simulink library "vhit_control_library"  (R2023a)
settings: Solver=VariableStepAuto  StartTime=0.0  StopTime=10.0  RelTol=1e-3
undefined symbols (not defined in the file): bit, cstElctSpdMaxVal, cstSlowTaskSampTime, parDirCurrMaxVal, parElctSpdMaxVal, parFluxObsFiltCoef, parQdrtCurrMaxVal, parRefSpdFallSlewRate, parRefSpdRisSlewRate, PolePairNum
libraries: lib_conversion x90, lib_square_root x11, lib_dynamic_saturator x9, lib_resettable_unit_delay x2, lib_fault_definiteness x1, lib_angle_mapper x1, lib_cart_to_polar_coor_transformer x1, lib_clarke_transform x1, lib_configurable_parameter x1, lib_current_control_decoupling x1, lib_derating_reference_speed_limiter x1, lib_discrete_time_integrator x1
(part 2 of 3)

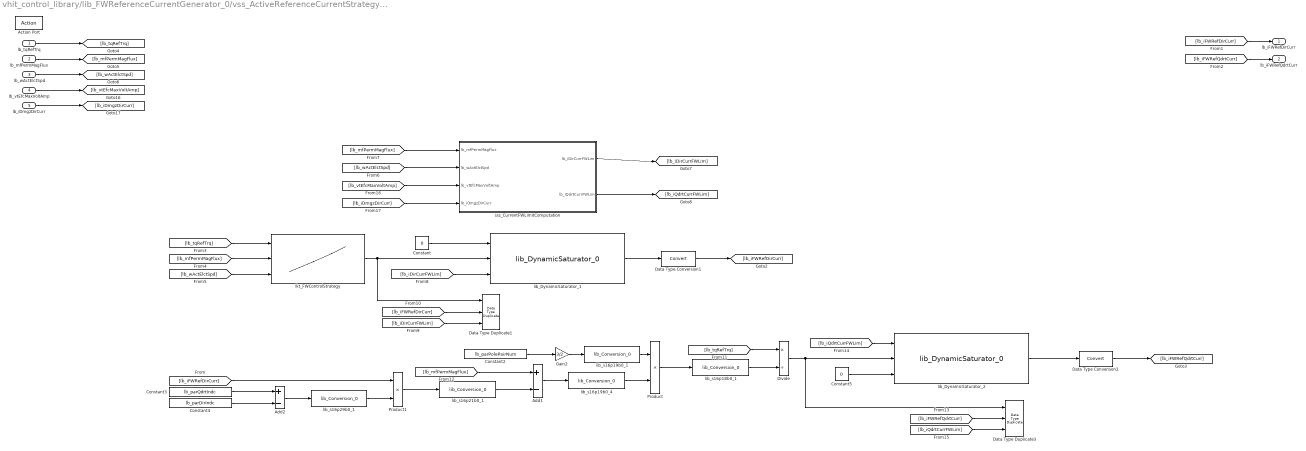
== system vhit_control_library/lib_FWReferenceCurrentGenerator_0/vss_ActiveReferenceCurrentStrategy/vss_FieldWeakeningStrategy/ias_FWControlStrategy ==
  lb_tqRefTrq : Inport
  lb_mfPermMagFlux : Inport  Port=2
  lb_wActElctSpd : Inport  Port=3
  lb_vtEfcMaxVoltAmp : Inport  Port=4
  lb_iDmgzDirCurr : Inport  Port=5
  Action Port : ActionPort
  Add1 : Sum  Inputs=+-  OutDataTypeStr=Inherit: Inherit via back propagation
  Add2 : Sum  Inputs=+-  OutDataTypeStr=Inherit: Inherit via back propagation
  Constant : Constant  Value=0  OutDataTypeStr=Inherit: Inherit via back propagation
  Constant2 : Constant  Value=lb_parPolePairNum
  Constant3 : Constant  Value=lb_parQdrtIndc
  Constant4 : Constant  Value=lb_parDirIndc
  Constant5 : Constant  Value=0  OutDataTypeStr=Inherit: Inherit via back propagation
  Data Type Duplicate1 : DataTypeDuplicate  NumInputPorts=3
  Data Type Duplicate3 : DataTypeDuplicate  NumInputPorts=3
  Data Type Conversion1 : DataTypeConversion  SaturateOnIntegerOverflow=off  RndMeth=Floor
  Data Type Conversion2 : DataTypeConversion  SaturateOnIntegerOverflow=off  RndMeth=Floor
  Divide : Product  Inputs=*/  OutDataTypeStr=Inherit: Inherit via back propagation
  Gain2 : Gain  Gain=3/2  OutDataTypeStr=Inherit: Inherit via back propagation
  Product : Product  OutDataTypeStr=Inherit: Inherit via back propagation
  Product1 : Product  OutDataTypeStr=Inherit: Inherit via back propagation
  lib_DynamicSaturator_1 : lib_dynamic_saturator/lib_DynamicSaturator_0
  lib_DynamicSaturator_2 : lib_dynamic_saturator/lib_DynamicSaturator_0
  lib_s16p18b0_1 : lib_conversion/lib_Conversion_0  lb_parDataType=fixdt(1,16,2^-18,0)  lb_parOutpMaxVal=[]  lb_parOutpMinVal=[]  lb_parSatFlag=off
  lib_s16p19b0_1 : lib_conversion/lib_Conversion_0  lb_parDataType=fixdt(0,16,10^-3,0)  lb_parOutpMaxVal=[]  lb_parOutpMinVal=[]  lb_parSatFlag=off
  lib_s16p19b0_4 : lib_conversion/lib_Conversion_0  lb_parDataType=fixdt(1,16,2^-19,0)  lb_parOutpMaxVal=[]  lb_parOutpMinVal=[]  lb_parSatFlag=off
  lib_s16p21b0_1 : lib_conversion/lib_Conversion_0  lb_parDataType=fixdt(1,16,2^-21,0)  lb_parOutpMaxVal=[]  lb_parOutpMinVal=[]  lb_parSatFlag=off
  lib_s16p29b0_1 : lib_conversion/lib_Conversion_0  lb_parDataType=fixdt(1,16,2^-29,0)  lb_parOutpMaxVal=[]  lb_parOutpMinVal=[]  lb_parSatFlag=off
  lkt_FWControlStrategy : Lookup_n-D  NumberOfTableDimensions=3  BreakpointsForDimension1=lb_parFWTrqData  BreakpointsForDimension2=lb_parFWPermMagFluxData  BreakpointsForDimension3=lb_parFWElctSpdData  BeginIndexSearchUsingPreviousIndexResult=on  Table=lb_parFW3DLktMtrx  ExtrapMethod=Clip  InternalRulePriority=Speed  OutDataTypeStr=Inherit: Inherit via back propagation  RndMeth=Simplest  InputSameDT=off
      settings: InputPortMap=u0,u1,u2
  sss_CurrentFWLimitComputation : Subsystem
  lb_iFWRefDirCurr : Outport
  lb_iFWRefQdrtCurr : Outport  Port=2
  wires:
  Constant2/1 -> Gain2/1
  Gain2/1 -> lib_s16p19b0_1/1
  lib_s16p19b0_1/1 -> Product/1
  [lb_wActElctSpd] -> sss_CurrentFWLimitComputation/2(lb_wActElctSpd)
  sss_CurrentFWLimitComputation/2(lb_iQdrtCurrFWLim) -> [lb_iQdrtCurrFWLim]
  [lb_mfPermMagFlux] -> sss_CurrentFWLimitComputation/1(lb_mfPermMagFlux)
  sss_CurrentFWLimitComputation/1(lb_iDirCurrFWLim) -> [lb_iDirCurrFWLim]
  Constant/1 -> lib_DynamicSaturator_1/1
  [lb_iDirCurrFWLim] -> lib_DynamicSaturator_1/3
  [lb_iFWRefDirCurr] -> lb_iFWRefDirCurr/1
  [lb_iFWRefQdrtCurr] -> lb_iFWRefQdrtCurr/1
  lb_mfPermMagFlux/1 -> [lb_mfPermMagFlux]
  lb_tqRefTrq/1 -> [lb_tqRefTrq]
  lb_wActElctSpd/1 -> [lb_wActElctSpd]
  [lb_tqRefTrq] -> lkt_FWControlStrategy/1
  [lb_mfPermMagFlux] -> lkt_FWControlStrategy/2
  [lb_wActElctSpd] -> lkt_FWControlStrategy/3
  lkt_FWControlStrategy/1 -> Data Type Duplicate1/1, lib_DynamicSaturator_1/2
  [lb_iFWRefDirCurr] -> Data Type Duplicate1/2
  [lb_iQdrtCurrFWLim] -> Data Type Duplicate3/3
  Constant5/1 -> lib_DynamicSaturator_2/3
  [lb_iQdrtCurrFWLim] -> lib_DynamicSaturator_2/1
  Data Type Conversion2/1 -> [lb_iFWRefQdrtCurr]
  lib_DynamicSaturator_2/1 -> Data Type Conversion2/1
  [lb_iFWRefQdrtCurr] -> Data Type Duplicate3/2
  Divide/1 -> Data Type Duplicate3/1, lib_DynamicSaturator_2/2
  [lb_iFWRefDirCurr] -> Product1/1
  lib_s16p19b0_4/1 -> Product/2
  Add1/1 -> lib_s16p19b0_4/1
  Add2/1 -> lib_s16p29b0_1/1
  Constant4/1 -> Add2/2
  Constant3/1 -> Add2/1
  Product1/1 -> lib_s16p21b0_1/1
  lib_s16p18b0_1/1 -> Divide/2
  [lb_mfPermMagFlux] -> Add1/1
  lib_s16p29b0_1/1 -> Product1/2
  Product/1 -> lib_s16p18b0_1/1
  lib_s16p21b0_1/1 -> Add1/2
  [lb_tqRefTrq] -> Divide/1
  lib_DynamicSaturator_1/1 -> Data Type Conversion1/1
  Data Type Conversion1/1 -> [lb_iFWRefDirCurr]
  [lb_iDirCurrFWLim] -> Data Type Duplicate1/3
  lb_vtEfcMaxVoltAmp/1 -> [lb_vtEfcMaxVoltAmp]
  lb_iDmgzDirCurr/1 -> [lb_iDmgzDirCurr]
  [lb_vtEfcMaxVoltAmp] -> sss_CurrentFWLimitComputation/3(lb_vtEfcMaxVoltAmp)
  [lb_iDmgzDirCurr] -> sss_CurrentFWLimitComputation/4(lb_iDmgzDirCurr)

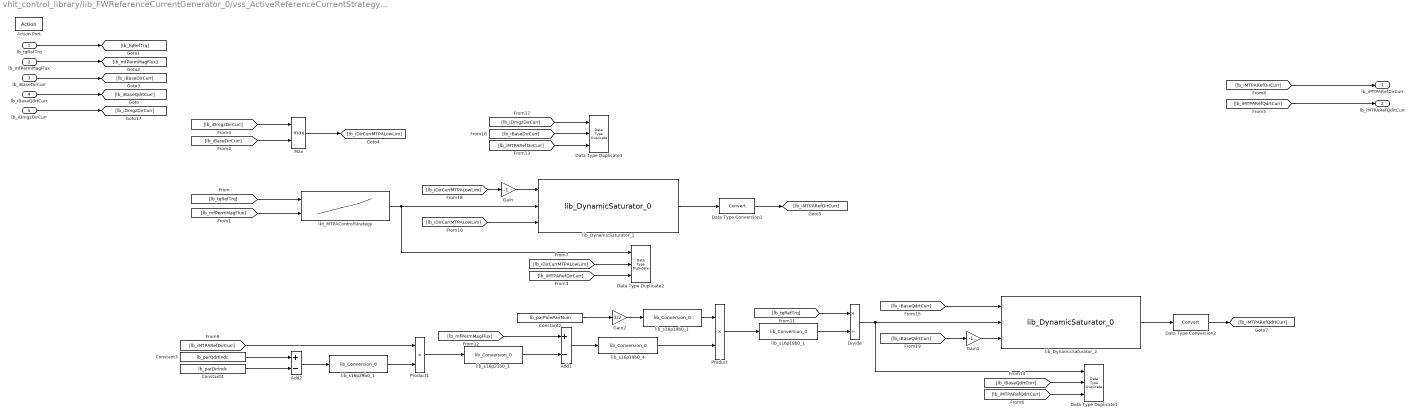
== system vhit_control_library/lib_FWReferenceCurrentGenerator_0/vss_ActiveReferenceCurrentStrategy/vss_FieldWeakeningStrategy/ias_MTPAControlStrategy ==
  lb_tqRefTrq : Inport
  lb_mfPermMagFlux : Inport  Port=2
  lb_iBaseDirCurr : Inport  Port=3
  lb_iBaseQdrtCurr : Inport  Port=4
  lb_iDmgzDirCurr : Inport  Port=5
  Action Port : ActionPort
  Add1 : Sum  Inputs=+-  OutDataTypeStr=Inherit: Inherit via back propagation
  Add2 : Sum  Inputs=+-  OutDataTypeStr=Inherit: Inherit via back propagation
  Constant2 : Constant  Value=lb_parPolePairNum
  Constant3 : Constant  Value=lb_parQdrtIndc
  Constant4 : Constant  Value=lb_parDirIndc
  Data Type Duplicate1 : DataTypeDuplicate  NumInputPorts=3
  Data Type Duplicate2 : DataTypeDuplicate  NumInputPorts=3
  Data Type Duplicate3 : DataTypeDuplicate  NumInputPorts=3
  Data Type Conversion1 : DataTypeConversion  SaturateOnIntegerOverflow=off  RndMeth=Floor
  Data Type Conversion2 : DataTypeConversion  SaturateOnIntegerOverflow=off  RndMeth=Floor
  Divide : Product  Inputs=*/  OutDataTypeStr=Inherit: Inherit via back propagation
  Gain : Gain  Gain=-1  OutDataTypeStr=Inherit: Inherit via back propagation
  Gain1 : Gain  Gain=-1  OutDataTypeStr=Inherit: Inherit via back propagation
  Gain2 : Gain  Gain=3/2  OutDataTypeStr=Inherit: Inherit via back propagation
  Max : MinMax  Function=max  Inputs=2  OutDataTypeStr=Inherit: Inherit via back propagation
  Product : Product  OutDataTypeStr=Inherit: Inherit via back propagation
  Product1 : Product  OutDataTypeStr=Inherit: Inherit via back propagation
  lib_DynamicSaturator_1 : lib_dynamic_saturator/lib_DynamicSaturator_0
  lib_DynamicSaturator_2 : lib_dynamic_saturator/lib_DynamicSaturator_0
  lib_s16p18b0_1 : lib_conversion/lib_Conversion_0  lb_parDataType=fixdt(1,16,2^-18,0)  lb_parOutpMaxVal=[]  lb_parOutpMinVal=[]  lb_parSatFlag=off
  lib_s16p19b0_1 : lib_conversion/lib_Conversion_0  lb_parDataType=fixdt(0,16,10^-3,0)  lb_parOutpMaxVal=[]  lb_parOutpMinVal=[]  lb_parSatFlag=off
  lib_s16p19b0_4 : lib_conversion/lib_Conversion_0  lb_parDataType=fixdt(1,16,2^-19,0)  lb_parOutpMaxVal=[]  lb_parOutpMinVal=[]  lb_parSatFlag=off
  lib_s16p21b0_1 : lib_conversion/lib_Conversion_0  lb_parDataType=fixdt(1,16,2^-21,0)  lb_parOutpMaxVal=[]  lb_parOutpMinVal=[]  lb_parSatFlag=off
  lib_s16p29b0_1 : lib_conversion/lib_Conversion_0  lb_parDataType=fixdt(1,16,2^-29,0)  lb_parOutpMaxVal=[]  lb_parOutpMinVal=[]  lb_parSatFlag=off
  lkt_MTPAControlStrategy : Lookup_n-D  BreakpointsForDimension1=lb_parMTPATrqData  BreakpointsForDimension2=lb_parMTPAPermMagFluxData  BeginIndexSearchUsingPreviousIndexResult=on  Table=lb_parMTPA2DLktMtrx  ExtrapMethod=Clip  InternalRulePriority=Speed  OutDataTypeStr=Inherit: Inherit via back propagation  RndMeth=Simplest  SaturateOnIntegerOverflow=on  InputSameDT=off
      settings: InputPortMap=u0,u1
  lb_iMTPARefDirCurr : Outport
  lb_iMTPARefQdrtCurr : Outport  Port=2
  wires:
  lib_s16p19b0_1/1 -> Product/1
  Gain2/1 -> lib_s16p19b0_1/1
  lb_tqRefTrq/1 -> [lb_tqRefTrq]
  lb_mfPermMagFlux/1 -> [lb_mfPermMagFlux]
  [lb_tqRefTrq] -> lkt_MTPAControlStrategy/1
  [lb_mfPermMagFlux] -> lkt_MTPAControlStrategy/2
  lkt_MTPAControlStrategy/1 -> lib_DynamicSaturator_1/2, Data Type Duplicate2/1
  [lb_iDirCurrMTPALowLim] -> Gain/1
  lib_DynamicSaturator_1/1 -> Data Type Conversion1/1
  [lb_iMTPARefDirCurr] -> lb_iMTPARefDirCurr/1
  [lb_iMTPARefQdrtCurr] -> lb_iMTPARefQdrtCurr/1
  Data Type Conversion1/1 -> [lb_iMTPARefDirCurr]
  [lb_iMTPARefDirCurr] -> Data Type Duplicate2/3
  [lb_iDirCurrMTPALowLim] -> Data Type Duplicate2/2
  Product/1 -> lib_s16p18b0_1/1
  lib_s16p19b0_4/1 -> Product/2
  Add1/1 -> lib_s16p19b0_4/1
  lib_s16p21b0_1/1 -> Add1/2
  lib_s16p18b0_1/1 -> Divide/2
  lib_s16p29b0_1/1 -> Product1/2
  Product1/1 -> lib_s16p21b0_1/1
  [lb_tqRefTrq] -> Divide/1
  [lb_mfPermMagFlux] -> Add1/1
  [lb_iMTPARefDirCurr] -> Product1/1
  Constant3/1 -> Add2/1
  Constant2/1 -> Gain2/1
  Constant4/1 -> Add2/2
  Add2/1 -> lib_s16p29b0_1/1
  [lb_iBaseQdrtCurr] -> Gain1/1
  Data Type Conversion2/1 -> [lb_iMTPARefQdrtCurr]
  lib_DynamicSaturator_2/1 -> Data Type Conversion2/1
  [lb_iBaseQdrtCurr] -> lib_DynamicSaturator_2/1
  Divide/1 -> lib_DynamicSaturator_2/2, Data Type Duplicate1/1
  lb_iBaseDirCurr/1 -> [lb_iBaseDirCurr]
  lb_iBaseQdrtCurr/1 -> [lb_iBaseQdrtCurr]
  [lb_iMTPARefQdrtCurr] -> Data Type Duplicate1/3
  [lb_iBaseQdrtCurr] -> Data Type Duplicate1/2
  lb_iDmgzDirCurr/1 -> [lb_iDmgzDirCurr]
  [lb_iBaseDirCurr] -> Max/2
  [lb_iDmgzDirCurr] -> Max/1
  Max/1 -> [lb_iDirCurrMTPALowLim]
  [lb_iDirCurrMTPALowLim] -> lib_DynamicSaturator_1/3
  [lb_iMTPARefDirCurr] -> Data Type Duplicate3/3
  [lb_iBaseDirCurr] -> Data Type Duplicate3/2
  [lb_iDmgzDirCurr] -> Data Type Duplicate3/1
  Gain/1 -> lib_DynamicSaturator_1/1
  Gain1/1 -> lib_DynamicSaturator_2/3

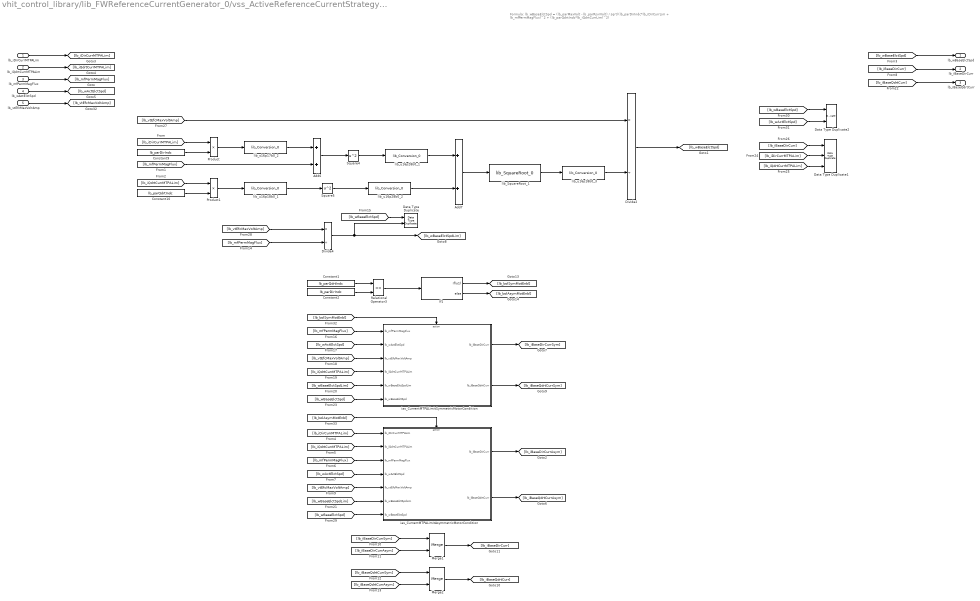
== system vhit_control_library/lib_FWReferenceCurrentGenerator_0/vss_ActiveReferenceCurrentStrategy/vss_FieldWeakeningStrategy/sss_BaseSpeedComputation ==
  note: Formula: lb_wBaseElctSpd = (lb_parMaxVolt - lb_parRsvrVolt) / sqrt((lb_parDirIndc*lb_iDirCurrLim + lb_mfPermMagFlux)^2 + (lb_parQdrtIndc*lb_iQdrtCurrLim)^2)
  lb_iDirCurrMTPALim : Inport
  lb_iQdrtCurrMTPALim : Inport  Port=2
  lb_mfPermMagFlux : Inport  Port=3
  lb_wActElctSpd : Inport  Port=4
  lb_vtEfcMaxVoltAmp : Inport  Port=5
  Add6 : Sum  OutDataTypeStr=Inherit: Same as first input
  Add7 : Sum  OutDataTypeStr=Inherit: Same as first input
  Constant1 : Constant  Value=lb_parQdrtIndc
  Constant10 : Constant  Value=lb_parQdrtIndc
  Constant2 : Constant  Value=lb_parDirIndc
  Constant9 : Constant  Value=lb_parDirIndc
  Data Type Duplicate : DataTypeDuplicate
  Data Type Duplicate1 : DataTypeDuplicate  NumInputPorts=3
  Data Type Duplicate2 : DataTypeDuplicate
  Divide2 : Product  Inputs=*/  OutDataTypeStr=Inherit: Inherit via back propagation
  Divide4 : Product  Inputs=*/  OutDataTypeStr=Inherit: Inherit via back propagation
  If1 : If  IfExpression=u1
  Merge1 : Merge
  Merge2 : Merge
  Product : Product  OutDataTypeStr=Inherit: Inherit via back propagation
  Product1 : Product  OutDataTypeStr=Inherit: Inherit via back propagation
  Relational Operator3 : RelationalOperator  Operator===  OutDataTypeStr=boolean  RndMeth=Simplest  InputSameDT=off
  Square4 : Math  Operator=square  SignedPower=on  OutDataTypeStr=Inherit: Inherit via back propagation
  Square5 : Math  Operator=square  SignedPower=on  OutDataTypeStr=Inherit: Inherit via back propagation
  ias_CurrentMTPALimitAsymmetricMotorCondition : Subsystem  TreatAsAtomicUnit=on
  ias_CurrentMTPALimitSymmetricMotorCondition : Subsystem  TreatAsAtomicUnit=on
  lib_SquareRoot_1 : lib_square_root/lib_SquareRoot_0  lb_parLktSize=128  lb_parInpDataType=uint16  lb_parOutpDataType=Inherit: Inherit via back propagation
  lib_s16p17b0_2 : lib_conversion/lib_Conversion_0  lb_parDataType=fixdt(1,16,2^-17,0)  lb_parOutpMaxVal=[]  lb_parOutpMinVal=[]  lb_parSatFlag=off
  lib_u16p18b0_1 : lib_conversion/lib_Conversion_0  lb_parDataType=fixdt(0,16,2^-18,0)  lb_parOutpMaxVal=[]  lb_parOutpMinVal=[]  lb_parSatFlag=off
  lib_u16p18b0_3 : lib_conversion/lib_Conversion_0  lb_parDataType=fixdt(0,16,2^-18,0)  lb_parOutpMaxVal=[]  lb_parOutpMinVal=[]  lb_parSatFlag=off
  lib_u16p28b0_1 : lib_conversion/lib_Conversion_0  lb_parDataType=fixdt(0,16,2^-28,0)  lb_parOutpMaxVal=[]  lb_parOutpMinVal=[]  lb_parSatFlag=off
  lib_u16p28b0_2 : lib_conversion/lib_Conversion_0  lb_parDataType=fixdt(0,16,2^-28,0)  lb_parOutpMaxVal=[]  lb_parOutpMinVal=[]  lb_parSatFlag=off
  lb_wBaseElctSpd : Outport
  lb_iBaseDirCurr : Outport  Port=2
  lb_iBaseQdrtCurr : Outport  Port=3
  wires:
  [lb_wBaseElctSpd] -> ias_CurrentMTPALimitAsymmetricMotorCondition/7(lb_wBaseElctSpd)
  [lb_wBaseElctSpd] -> ias_CurrentMTPALimitSymmetricMotorCondition/6(lb_wBaseElctSpd)
  [lb_wBaseElctSpdLim] -> ias_CurrentMTPALimitAsymmetricMotorCondition/6(lb_wBaseElctSpdLim)
  [lb_wBaseElctSpdLim] -> ias_CurrentMTPALimitSymmetricMotorCondition/5(lb_wBaseElctSpdLim)
  [lb_iQdrtCurrMTPALim] -> ias_CurrentMTPALimitSymmetricMotorCondition/4(lb_iQdrtCurrMTPALim)
  [lb_vtEfcMaxVoltAmp] -> ias_CurrentMTPALimitSymmetricMotorCondition/3(lb_vtEfcMaxVoltAmp)
  [lb_wActElctSpd] -> ias_CurrentMTPALimitSymmetricMotorCondition/2(lb_wActElctSpd)
  [lb_mfPermMagFlux] -> ias_CurrentMTPALimitSymmetricMotorCondition/1(lb_mfPermMagFlux)
  Merge2/1 -> [lb_iBaseQdrtCurr]
  [lb_iBaseQdrtCurrAsym] -> Merge2/2
  [lb_iBaseQdrtCurrSym] -> Merge2/1
  ias_CurrentMTPALimitSymmetricMotorCondition/2(lb_iBaseQdrtCurr) -> [lb_iBaseQdrtCurrSym]
  ias_CurrentMTPALimitSymmetricMotorCondition/1(lb_iBaseDirCurr) -> [lb_iBaseDirCurrSym]
  [lb_vtEfcMaxVoltAmp] -> ias_CurrentMTPALimitAsymmetricMotorCondition/5(lb_vtEfcMaxVoltAmp)
  [lb_wActElctSpd] -> ias_CurrentMTPALimitAsymmetricMotorCondition/4(lb_wActElctSpd)
  [lb_mfPermMagFlux] -> ias_CurrentMTPALimitAsymmetricMotorCondition/3(lb_mfPermMagFlux)
  [lb_iQdrtCurrMTPALim] -> ias_CurrentMTPALimitAsymmetricMotorCondition/2(lb_iQdrtCurrMTPALim)
  [lb_iDirCurrMTPALim] -> ias_CurrentMTPALimitAsymmetricMotorCondition/1(lb_iDirCurrMTPALim)
  [lb_bolSymMotEnbl] -> ias_CurrentMTPALimitSymmetricMotorCondition/Action
  ias_CurrentMTPALimitAsymmetricMotorCondition/2(lb_iBaseQdrtCurr) -> [lb_iBaseQdrtCurrAsym]
  Constant2/1 -> Relational Operator3/2
  If1/2 -> [lb_bolAsymMotEnbl]
  If1/1 -> [lb_bolSymMotEnbl]
  ias_CurrentMTPALimitAsymmetricMotorCondition/1(lb_iBaseDirCurr) -> [lb_iBaseDirCurrAsym]
  Constant1/1 -> Relational Operator3/1
  [lb_iBaseDirCurrAsym] -> Merge1/2
  [lb_bolAsymMotEnbl] -> ias_CurrentMTPALimitAsymmetricMotorCondition/Action
  [lb_iBaseDirCurrSym] -> Merge1/1
  Relational Operator3/1 -> If1/1
  Merge1/1 -> [lb_iBaseDirCurr]
  lb_iQdrtCurrMTPALim/1 -> [lb_iQdrtCurrMTPALim]
  lb_iDirCurrMTPALim/1 -> [lb_iDirCurrMTPALim]
  lb_mfPermMagFlux/1 -> [lb_mfPermMagFlux]
  [lb_wBaseElctSpd] -> lb_wBaseElctSpd/1
  Square5/1 -> lib_u16p28b0_2/1
  Square4/1 -> lib_u16p28b0_1/1
  lib_u16p28b0_1/1 -> Add7/1
  lib_u16p18b0_3/1 -> Divide2/2
  lib_s16p17b0_2/1 -> Add6/1
  Add7/1 -> lib_SquareRoot_1/1
  Constant9/1 -> Product/2
  Divide2/1 -> [lb_wBaseElctSpd]
  [lb_vtEfcMaxVoltAmp] -> Divide2/1
  [lb_iQdrtCurrMTPALim] -> Product1/1
  lib_u16p28b0_2/1 -> Add7/2
  Add6/1 -> Square4/1
  Constant10/1 -> Product1/2
  [lb_mfPermMagFlux] -> Add6/2
  [lb_iDirCurrMTPALim] -> Product/1
  Product1/1 -> lib_u16p18b0_1/1
  lib_SquareRoot_1/1 -> lib_u16p18b0_3/1
  lib_u16p18b0_1/1 -> Square5/1
  Product/1 -> lib_s16p17b0_2/1
  [lb_iBaseDirCurr] -> lb_iBaseDirCurr/1
  lb_wActElctSpd/1 -> [lb_wActElctSpd]
  [lb_mfPermMagFlux] -> Divide4/2
  Divide4/1 -> Data Type Duplicate/2, [lb_wBaseElctSpdLim]
  [lb_wBaseElctSpd] -> Data Type Duplicate/1
  [lb_iBaseQdrtCurr] -> lb_iBaseQdrtCurr/1
  [lb_iBaseDirCurr] -> Data Type Duplicate1/1
  [lb_iDirCurrMTPALim] -> Data Type Duplicate1/2
  [lb_iQdrtCurrMTPALim] -> Data Type Duplicate1/3
  lb_vtEfcMaxVoltAmp/1 -> [lb_vtEfcMaxVoltAmp]
  [lb_vtEfcMaxVoltAmp] -> Divide4/1
  [lb_wBaseElctSpd] -> Data Type Duplicate2/1
  [lb_wActElctSpd] -> Data Type Duplicate2/2

== system vhit_control_library/lib_FWReferenceCurrentGenerator_0/vss_ActiveReferenceCurrentStrategy/vss_FieldWeakeningStrategy/sss_CurrentMTPALimitComputation ==
  note: Formula:
      | lb_iDirCurrMTPALim = lb_mfPermMagFlux/4/(lb_parQdrtIndc-lb_parDirIndc) - sqrt((lb_mfPermMagFlux/4/(lb_parQdrtIndc-lb_parDirIndc))^2 + 1/2*lb_parMaxPhsCurr^2
      | lb_iQdrtCurrMTPALim = sqrt(lb_parMaxPhsCurr^2 - lb_iDirCurrMTPALim^2)
  lb_mfPermMagFlux : Inport
  Constant1 : Constant  Value=lb_parQdrtIndc
  Constant2 : Constant  Value=lb_parDirIndc
  If : If  IfExpression=u1
  Merge : Merge
  Merge1 : Merge
  Relational Operator : RelationalOperator  Operator===  OutDataTypeStr=boolean  RndMeth=Simplest  InputSameDT=off
  ias_CurrentMTPALimitAsymmetricMotorCondition : Subsystem  TreatAsAtomicUnit=on
  ias_CurrentMTPALimitSymmetricMotorCondition : Subsystem  TreatAsAtomicUnit=on
  lb_iDirCurrMTPALim : Outport
  lb_iQdrtCurrMTPALim : Outport  Port=2
  wires:
  Merge1/1 -> [lb_iQdrtCurrMTPALim]
  Merge/1 -> [lb_iDirCurrMTPALim]
  [lb_iQdrtCurrMTPALimAsym] -> Merge1/2
  [lb_iQdrtCurrMTPALimSym] -> Merge1/1
  [lb_iDirCurrMTPALimSym] -> Merge/1
  [lb_iDirCurrMTPALimAsym] -> Merge/2
  [lb_mfPermMagFlux] -> ias_CurrentMTPALimitAsymmetricMotorCondition/1(lb_mfPermMagFlux)
  ias_CurrentMTPALimitAsymmetricMotorCondition/2(lb_iQdrtCurrMTPALim) -> [lb_iQdrtCurrMTPALimAsym]
  ias_CurrentMTPALimitAsymmetricMotorCondition/1(lb_iDirCurrMTPALim) -> [lb_iDirCurrMTPALimAsym]
  ias_CurrentMTPALimitSymmetricMotorCondition/2(lb_iQdrtCurrMTPALim) -> [lb_iQdrtCurrMTPALimSym]
  ias_CurrentMTPALimitSymmetricMotorCondition/1(lb_iDirCurrMTPALim) -> [lb_iDirCurrMTPALimSym]
  [lb_bolAsymMotEnbl] -> ias_CurrentMTPALimitAsymmetricMotorCondition/Action
  [lb_bolSymMotEnbl] -> ias_CurrentMTPALimitSymmetricMotorCondition/Action
  If/2 -> [lb_bolAsymMotEnbl]
  If/1 -> [lb_bolSymMotEnbl]
  Relational Operator/1 -> If/1
  Constant2/1 -> Relational Operator/2
  Constant1/1 -> Relational Operator/1
  [lb_iDirCurrMTPALim] -> lb_iDirCurrMTPALim/1
  [lb_iQdrtCurrMTPALim] -> lb_iQdrtCurrMTPALim/1
  lb_mfPermMagFlux/1 -> [lb_mfPermMagFlux]

== system vhit_control_library/lib_FWReferenceCurrentGenerator_0/vss_ActiveReferenceCurrentStrategy/vss_FieldWeakeningStrategy/sss_DemagnetizationCurrentComputation ==
  lb_mfPermMagFlux : Inport
  Constant : Constant  Value=lb_parDmgzFact
  Constant1 : Constant  Value=lb_parDirIndc
  Data Type Duplicate : DataTypeDuplicate
  Divide3 : Product  Inputs=*/  OutDataTypeStr=Inherit: Inherit via back propagation
  Gain : Gain  Gain=-1  OutDataTypeStr=Inherit: Inherit via back propagation
  Product2 : Product  OutDataTypeStr=Inherit: Same as first input
  lb_iDmgzLimRefDirCurr : Outport
  wires:
  Divide3/1 -> Gain/1, Data Type Duplicate/1
  Product2/1 -> Divide3/1
  [lb_mfPermMagFlux] -> Product2/1
  Gain/1 -> [lb_iDmgzLimRefDirCurr], Data Type Duplicate/2
  Constant/1 -> Product2/2
  lb_mfPermMagFlux/1 -> [lb_mfPermMagFlux]
  [lb_iDmgzLimRefDirCurr] -> lb_iDmgzLimRefDirCurr/1
  Constant1/1 -> Divide3/2

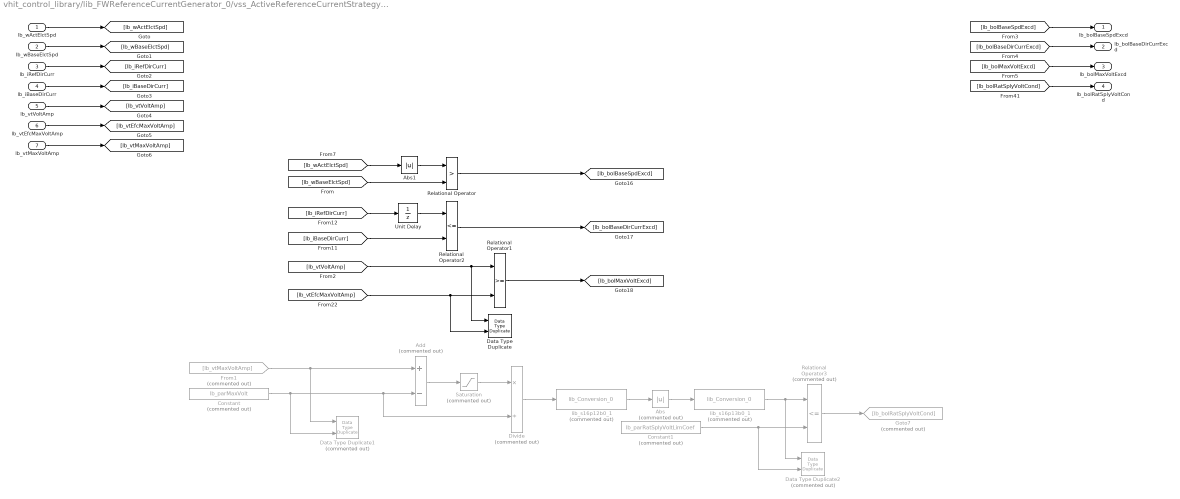
== system vhit_control_library/lib_FWReferenceCurrentGenerator_0/vss_ActiveReferenceCurrentStrategy/vss_FieldWeakeningStrategy/sss_MTPAAndFWTransitionCondition ==
  lb_wActElctSpd : Inport
  lb_wBaseElctSpd : Inport  Port=2
  lb_iRefDirCurr : Inport  Port=3
  lb_iBaseDirCurr : Inport  Port=4
  lb_vtVoltAmp : Inport  Port=5
  lb_vtEfcMaxVoltAmp : Inport  Port=6
  lb_vtMaxVoltAmp : Inport  Port=7
  Abs : Abs  Commented=on  OutDataTypeStr=Inherit: Inherit via back propagation  SaturateOnIntegerOverflow=off
  Abs1 : Abs  SaturateOnIntegerOverflow=off
  Add : Sum  Commented=on  Inputs=+-  OutDataTypeStr=Inherit: Same as first input
  Constant : Constant  Commented=on  Value=lb_parMaxVolt  OutDataTypeStr=Inherit: Inherit via back propagation
  Constant1 : Constant  Commented=on  Value=lb_parRatSplyVoltLimCoef  OutDataTypeStr=Inherit: Inherit via back propagation
  Data Type Duplicate : DataTypeDuplicate
  Data Type Duplicate1 : DataTypeDuplicate  Commented=on
  Data Type Duplicate2 : DataTypeDuplicate  Commented=on
  Divide : Product  Commented=on  Inputs=*/  OutDataTypeStr=Inherit: Inherit via back propagation
  From1 : From  Commented=on  GotoTag=lb_vtMaxVoltAmp
  Goto7 : Goto  Commented=on  GotoTag=lb_bolRatSplyVoltCond
  Relational Operator : RelationalOperator  Operator=>  OutDataTypeStr=boolean  RndMeth=Simplest  InputSameDT=off
  Relational Operator1 : RelationalOperator  OutDataTypeStr=boolean  RndMeth=Simplest  InputSameDT=off
  Relational Operator2 : RelationalOperator  Operator=<=  OutDataTypeStr=boolean  RndMeth=Simplest  InputSameDT=off
  Relational Operator3 : RelationalOperator  Commented=on  Operator=<=  OutDataTypeStr=boolean  RndMeth=Simplest  InputSameDT=off
  Saturation : Saturate  Commented=on  UpperLimit=2*lb_parMaxVolt  LowerLimit=-2*lb_parMaxVolt
  Unit Delay : UnitDelay  SampleTime=-1  HasFrameUpgradeWarning=on
  lib_s16p12b0_1 : lib_conversion/lib_Conversion_0  Commented=on  lb_parDataType=Inherit: Inherit via back propagation  lb_parOutpMaxVal=[]  lb_parOutpMinVal=[]  lb_parSatFlag=off
  lib_s16p13b0_1 : lib_conversion/lib_Conversion_0  Commented=on  lb_parDataType=Inherit: Inherit via back propagation  lb_parOutpMaxVal=[]  lb_parOutpMinVal=[]  lb_parSatFlag=off
  lb_bolBaseSpdExcd : Outport
  lb_bolBaseDirCurrExcd : Outport  Port=2
  lb_bolMaxVoltExcd : Outport  Port=3
  lb_bolRatSplyVoltCond : Outport  Port=4
  wires:
  Relational Operator2/1 -> [lb_bolBaseDirCurrExcd]
  [lb_iRefDirCurr] -> Unit Delay/1
  Relational Operator/1 -> [lb_bolBaseSpdExcd]
  [lb_wActElctSpd] -> Abs1/1
  Unit Delay/1 -> Relational Operator2/1
  [lb_vtVoltAmp] -> Relational Operator1/1, Data Type Duplicate/1
  [lb_iBaseDirCurr] -> Relational Operator2/2
  [lb_vtEfcMaxVoltAmp] -> Relational Operator1/2, Data Type Duplicate/2
  Relational Operator1/1 -> [lb_bolMaxVoltExcd]
  [lb_wBaseElctSpd] -> Relational Operator/2
  lb_wActElctSpd/1 -> [lb_wActElctSpd]
  lb_wBaseElctSpd/1 -> [lb_wBaseElctSpd]
  lb_iRefDirCurr/1 -> [lb_iRefDirCurr]
  lb_iBaseDirCurr/1 -> [lb_iBaseDirCurr]
  lb_vtVoltAmp/1 -> [lb_vtVoltAmp]
  lb_vtEfcMaxVoltAmp/1 -> [lb_vtEfcMaxVoltAmp]
  lb_vtMaxVoltAmp/1 -> [lb_vtMaxVoltAmp]
  From1/1 -> Data Type Duplicate1/1, Add/1
  Constant/1 -> Data Type Duplicate1/2, Divide/2, Add/2
  Add/1 -> Saturation/1
  Saturation/1 -> Divide/1
  Divide/1 -> lib_s16p12b0_1/1
  lib_s16p12b0_1/1 -> Abs/1
  Abs/1 -> lib_s16p13b0_1/1
  lib_s16p13b0_1/1 -> Data Type Duplicate2/1, Relational Operator3/1
  Constant1/1 -> Data Type Duplicate2/2, Relational Operator3/2
  [lb_bolBaseSpdExcd] -> lb_bolBaseSpdExcd/1
  [lb_bolBaseDirCurrExcd] -> lb_bolBaseDirCurrExcd/1
  [lb_bolMaxVoltExcd] -> lb_bolMaxVoltExcd/1
  [lb_bolRatSplyVoltCond] -> lb_bolRatSplyVoltCond/1
  Relational Operator3/1 -> Goto7/1
  Abs1/1 -> Relational Operator/1

== system vhit_control_library/lib_FWReferenceCurrentGenerator_0/vss_ActiveReferenceCurrentStrategy/vss_FieldWeakeningStrategy/sss_MTPAAndFWTransitionLogic ==
  lb_bolBaseSpdExcd : Inport
  lb_bolBaseDirCurrExcd : Inport  Port=2
  lb_bolMaxVoltExcd : Inport  Port=3
  lb_bolRatSplyVoltCond : Inport  Port=4
  sfc_MTPAAndFWTransitionLogic : Stateflow chart  TreatAsAtomicUnit=on
  lb_bolFWCond : Outport
  wires:
  lb_bolBaseSpdExcd/1 -> sfc_MTPAAndFWTransitionLogic/1(lb_bolBaseSpdExcd)
  lb_bolBaseDirCurrExcd/1 -> sfc_MTPAAndFWTransitionLogic/2(lb_bolBaseDirCurrExcd)
  lb_bolMaxVoltExcd/1 -> sfc_MTPAAndFWTransitionLogic/3(lb_bolMaxVoltExcd)
  sfc_MTPAAndFWTransitionLogic/1(lb_bolFWCond) -> lb_bolFWCond/1
  lb_bolRatSplyVoltCond/1 -> sfc_MTPAAndFWTransitionLogic/4(lb_bolRatSplyVoltCond)

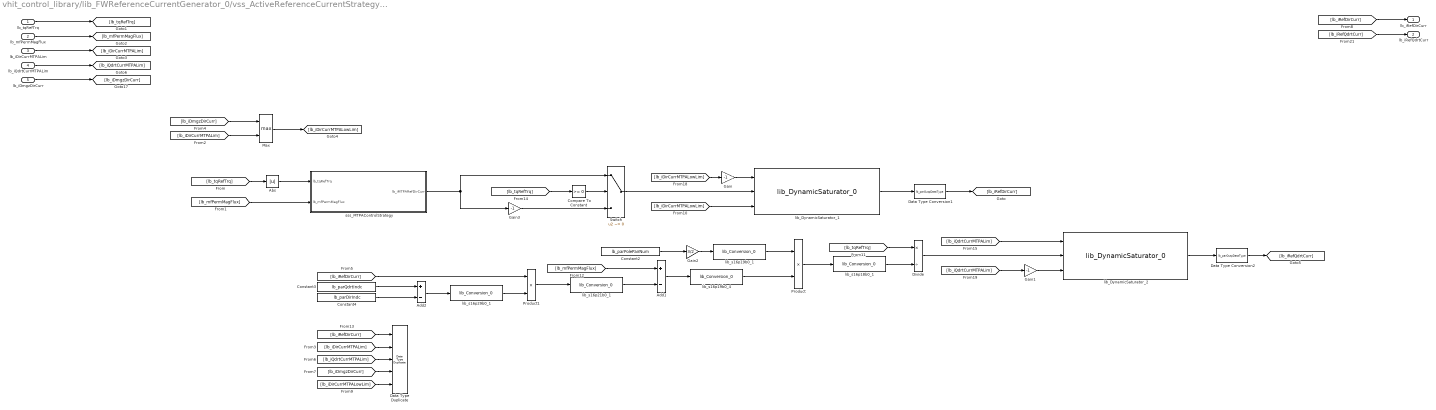
== system vhit_control_library/lib_FWReferenceCurrentGenerator_0/vss_ActiveReferenceCurrentStrategy/vss_MaximumTorquePerAmpereStrategy/ias_MTPAControlStrategy ==
  lb_tqRefTrq : Inport
  lb_mfPermMagFlux : Inport  Port=2
  lb_iDirCurrMTPALim : Inport  Port=3
  lb_iQdrtCurrMTPALim : Inport  Port=4
  lb_iDmgzDirCurr : Inport  Port=5
  Abs : Abs  SaturateOnIntegerOverflow=off
  Add1 : Sum  Inputs=+-  OutDataTypeStr=Inherit: Inherit via back propagation  RndMeth=Simplest
  Add2 : Sum  Inputs=+-  OutDataTypeStr=Inherit: Inherit via back propagation  RndMeth=Simplest
  Compare To Constant : simulink/Logic and Bit Operations/Compare To Constant  relop=>=  const=0  OutDataTypeStr=boolean
  Constant2 : Constant  Value=lb_parPolePairNum
  Constant3 : Constant  Value=lb_parQdrtIndc
  Constant4 : Constant  Value=lb_parDirIndc
  Data Type Duplicate : DataTypeDuplicate  NumInputPorts=5
  Data Type Conversion1 : DataTypeConversion  OutDataTypeStr=lb_parOutpDataType  SaturateOnIntegerOverflow=off  RndMeth=Floor
  Data Type Conversion2 : DataTypeConversion  OutDataTypeStr=lb_parOutpDataType  SaturateOnIntegerOverflow=off  RndMeth=Floor
  Divide : Product  Inputs=*/  OutDataTypeStr=Inherit: Inherit via back propagation  RndMeth=Simplest
  Gain : Gain  Gain=-1  OutDataTypeStr=Inherit: Inherit via back propagation  RndMeth=Simplest
  Gain1 : Gain  Gain=-1  OutDataTypeStr=Inherit: Inherit via back propagation  RndMeth=Simplest
  Gain2 : Gain  Gain=3/2  OutDataTypeStr=Inherit: Inherit via back propagation  RndMeth=Simplest
  Gain3 : Gain  Gain=-1  OutDataTypeStr=Inherit: Same as input
  Max : MinMax  Function=max  Inputs=2  OutDataTypeStr=Inherit: Inherit via back propagation
  Product : Product  OutDataTypeStr=Inherit: Inherit via back propagation  RndMeth=Simplest
  Product1 : Product  OutDataTypeStr=Inherit: Inherit via back propagation  RndMeth=Simplest
  Switch : Switch  Criteria=u2 ~= 0  SaturateOnIntegerOverflow=off  InputSameDT=off
  lib_DynamicSaturator_1 : lib_dynamic_saturator/lib_DynamicSaturator_0
  lib_DynamicSaturator_2 : lib_dynamic_saturator/lib_DynamicSaturator_0
  lib_s16p18b0_1 : lib_conversion/lib_Conversion_0  lb_parDataType=fixdt(1,16,2^-18,0)  lb_parOutpMaxVal=[]  lb_parOutpMinVal=[]  lb_parSatFlag=off
  lib_s16p19b0_1 : lib_conversion/lib_Conversion_0  lb_parDataType=fixdt(0,16,10^-3,0)  lb_parOutpMaxVal=[]  lb_parOutpMinVal=[]  lb_parSatFlag=off
  lib_s16p19b0_4 : lib_conversion/lib_Conversion_0  lb_parDataType=fixdt(1,16,2^-19,0)  lb_parOutpMaxVal=[]  lb_parOutpMinVal=[]  lb_parSatFlag=off
  lib_s16p21b0_1 : lib_conversion/lib_Conversion_0  lb_parDataType=fixdt(1,16,2^-21,0)  lb_parOutpMaxVal=[]  lb_parOutpMinVal=[]  lb_parSatFlag=off
  lib_s16p29b0_1 : lib_conversion/lib_Conversion_0  lb_parDataType=fixdt(1,16,2^-29,0)  lb_parOutpMaxVal=[]  lb_parOutpMinVal=[]  lb_parSatFlag=off
  sss_MTPAControlStrategy : Subsystem
  lb_iRefDirCurr : Outport
  lb_iRefQdrtCurr : Outport  Port=2
  wires:
  [lb_iRefDirCurr] -> Data Type Duplicate/1
  [lb_iDirCurrMTPALowLim] -> Data Type Duplicate/5
  [lb_iQdrtCurrMTPALim] -> Data Type Duplicate/3
  [lb_iDmgzDirCurr] -> Data Type Duplicate/4
  [lb_iDirCurrMTPALim] -> Data Type Duplicate/2
  [lb_iRefDirCurr] -> lb_iRefDirCurr/1
  [lb_iRefQdrtCurr] -> lb_iRefQdrtCurr/1
  lib_s16p19b0_1/1 -> Product/1
  Gain2/1 -> lib_s16p19b0_1/1
  lb_tqRefTrq/1 -> [lb_tqRefTrq]
  lb_mfPermMagFlux/1 -> [lb_mfPermMagFlux]
  [lb_tqRefTrq] -> Abs/1
  [lb_mfPermMagFlux] -> sss_MTPAControlStrategy/2(lb_mfPermMagFlux)
  [lb_iDirCurrMTPALowLim] -> Gain/1
  lib_DynamicSaturator_1/1 -> Data Type Conversion1/1
  Data Type Conversion1/1 -> [lb_iRefDirCurr]
  Product/1 -> lib_s16p18b0_1/1
  lib_s16p19b0_4/1 -> Product/2
  Add1/1 -> lib_s16p19b0_4/1
  lib_s16p21b0_1/1 -> Add1/2
  lib_s16p18b0_1/1 -> Divide/2
  lib_s16p29b0_1/1 -> Product1/2
  Product1/1 -> lib_s16p21b0_1/1
  [lb_tqRefTrq] -> Divide/1
  [lb_mfPermMagFlux] -> Add1/1
  [lb_iRefDirCurr] -> Product1/1
  Constant3/1 -> Add2/1
  Constant2/1 -> Gain2/1
  Constant4/1 -> Add2/2
  Add2/1 -> lib_s16p29b0_1/1
  [lb_iQdrtCurrMTPALim] -> Gain1/1
  Data Type Conversion2/1 -> [lb_iRefQdrtCurr]
  lib_DynamicSaturator_2/1 -> Data Type Conversion2/1
  [lb_iQdrtCurrMTPALim] -> lib_DynamicSaturator_2/1
  Divide/1 -> lib_DynamicSaturator_2/2
  lb_iDirCurrMTPALim/1 -> [lb_iDirCurrMTPALim]
  lb_iQdrtCurrMTPALim/1 -> [lb_iQdrtCurrMTPALim]
  lb_iDmgzDirCurr/1 -> [lb_iDmgzDirCurr]
  [lb_iDirCurrMTPALim] -> Max/2
  [lb_iDmgzDirCurr] -> Max/1
  Max/1 -> [lb_iDirCurrMTPALowLim]
  [lb_iDirCurrMTPALowLim] -> lib_DynamicSaturator_1/3
  Gain/1 -> lib_DynamicSaturator_1/1
  Gain1/1 -> lib_DynamicSaturator_2/3
  Abs/1 -> sss_MTPAControlStrategy/1(lb_tqRefTrq)
  [lb_tqRefTrq] -> Compare To Constant/1
  Compare To Constant/1 -> Switch/2
  Gain3/1 -> Switch/3
  Switch/1 -> lib_DynamicSaturator_1/2
  sss_MTPAControlStrategy/1(lb_iMTPARefDirCurr) -> Gain3/1, Switch/1

== system vhit_control_library/lib_FWReferenceCurrentGenerator_0/vss_ActiveReferenceCurrentStrategy/vss_MaximumTorquePerAmpereStrategy/sss_CurrentMTPALimitComputation ==
  note: Formula:
      | lb_iDirCurrMTPALim = lb_mfPermMagFlux/4/(lb_parQdrtIndc-lb_parDirIndc) - sqrt((lb_mfPermMagFlux/4/(lb_parQdrtIndc-lb_parDirIndc))^2 + 1/2*lb_parMaxPhsCurr^2
      | lb_iQdrtCurrMTPALim = sqrt(lb_parMaxPhsCurr^2 - lb_iDirCurrMTPALim^2)
  lb_mfPermMagFlux : Inport
  Constant1 : Constant  Value=lb_parQdrtIndc
  Constant2 : Constant  Value=lb_parDirIndc
  If : If  IfExpression=u1
  Merge : Merge
  Merge1 : Merge
  Relational Operator : RelationalOperator  Operator===  OutDataTypeStr=boolean  RndMeth=Simplest  InputSameDT=off
  ias_CurrentMTPALimitAsymmetricMotorCondition : Subsystem  TreatAsAtomicUnit=on
  ias_CurrentMTPALimitSymmetricMotorCondition : Subsystem  TreatAsAtomicUnit=on
  lb_iDirCurrMTPALim : Outport
  lb_iQdrtCurrMTPALim : Outport  Port=2
  wires:
  Merge1/1 -> [lb_iQdrtCurrMTPALim]
  Merge/1 -> [lb_iDirCurrMTPALim]
  [lb_iQdrtCurrMTPALimAsym] -> Merge1/2
  [lb_iQdrtCurrMTPALimSym] -> Merge1/1
  [lb_iDirCurrMTPALimSym] -> Merge/1
  [lb_iDirCurrMTPALimAsym] -> Merge/2
  [lb_mfPermMagFlux] -> ias_CurrentMTPALimitAsymmetricMotorCondition/1(lb_mfPermMagFlux)
  ias_CurrentMTPALimitAsymmetricMotorCondition/2(lb_iQdrtCurrMTPALim) -> [lb_iQdrtCurrMTPALimAsym]
  ias_CurrentMTPALimitAsymmetricMotorCondition/1(lb_iDirCurrMTPALim) -> [lb_iDirCurrMTPALimAsym]
  ias_CurrentMTPALimitSymmetricMotorCondition/2(lb_iQdrtCurrMTPALim) -> [lb_iQdrtCurrMTPALimSym]
  ias_CurrentMTPALimitSymmetricMotorCondition/1(lb_iDirCurrMTPALim) -> [lb_iDirCurrMTPALimSym]
  [lb_bolAsymMotEnbl] -> ias_CurrentMTPALimitAsymmetricMotorCondition/Action
  [lb_bolSymMotEnbl] -> ias_CurrentMTPALimitSymmetricMotorCondition/Action
  If/2 -> [lb_bolAsymMotEnbl]
  If/1 -> [lb_bolSymMotEnbl]
  Relational Operator/1 -> If/1
  Constant2/1 -> Relational Operator/2
  Constant1/1 -> Relational Operator/1
  [lb_iDirCurrMTPALim] -> lb_iDirCurrMTPALim/1
  [lb_iQdrtCurrMTPALim] -> lb_iQdrtCurrMTPALim/1
  lb_mfPermMagFlux/1 -> [lb_mfPermMagFlux]

== system vhit_control_library/lib_FWReferenceCurrentGenerator_0/vss_ActiveReferenceCurrentStrategy/vss_MaximumTorquePerAmpereStrategy/sss_DemagnetizationCurrentComputation ==
  lb_mfPermMagFlux : Inport
  Constant : Constant  Value=lb_parDmgzFact
  Constant1 : Constant  Value=lb_parDirIndc
  Data Type Duplicate : DataTypeDuplicate
  Divide3 : Product  Inputs=*/  OutDataTypeStr=Inherit: Inherit via back propagation  RndMeth=Simplest
  Gain : Gain  Gain=-1  OutDataTypeStr=Inherit: Inherit via back propagation  RndMeth=Simplest
  Product2 : Product  RndMeth=Simplest  OutDataTypeStr=Inherit: Same as first input
  lb_iDmgzLimRefDirCurr : Outport
  wires:
  Divide3/1 -> Gain/1, Data Type Duplicate/1
  Product2/1 -> Divide3/1
  [lb_mfPermMagFlux] -> Product2/1
  Gain/1 -> [lb_iDmgzLimRefDirCurr], Data Type Duplicate/2
  Constant/1 -> Product2/2
  lb_mfPermMagFlux/1 -> [lb_mfPermMagFlux]
  [lb_iDmgzLimRefDirCurr] -> lb_iDmgzLimRefDirCurr/1
  Constant1/1 -> Divide3/2

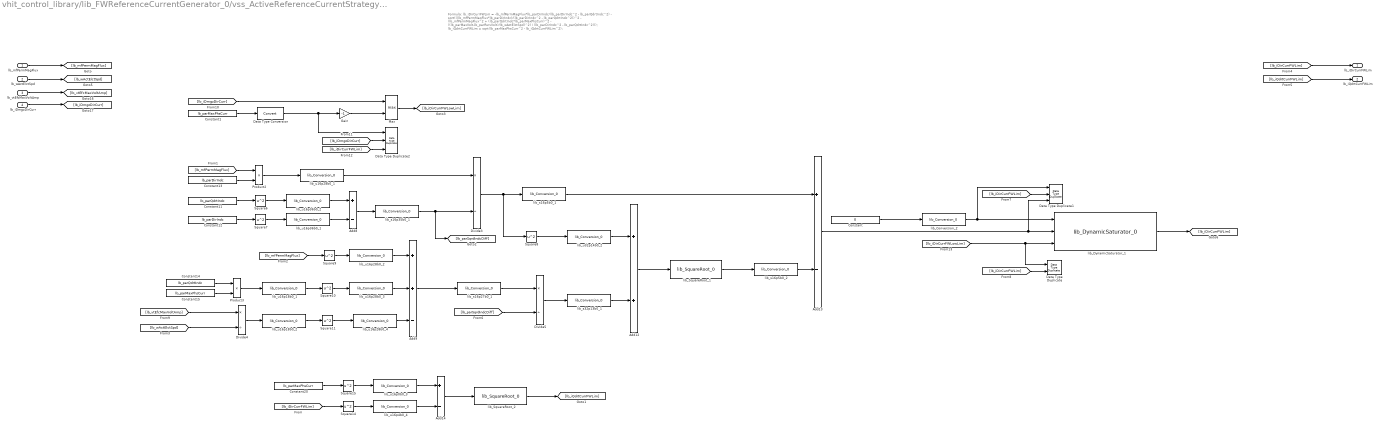
== system vhit_control_library/lib_FWReferenceCurrentGenerator_0/vss_ActiveReferenceCurrentStrategy/vss_FieldWeakeningStrategy/ias_FWControlStrategy/sss_CurrentFWLimitComputation ==
  note: Formula:
      | lb_iDirCurrFWLim = -lb_mfPermMagFlux*lb_parDirIndc/(lb_parDirIndc^2 - lb_parQdrtIndc^2) - sqrt(((lb_mfPermMagFlux*lb_parDirIndc)/(lb_parDirIndc^2 - lb_parQdrtIndc^2))^2 - (lb_mfPermMagFlux^2 + (lb_parQdrtIndc*lb_parMaxPhsCurr)^2 - ((lb_parMaxVolt-lb_parRsrvVolt)/lb_wActElctSpd)^2) / (lb_parDirIndc^2 - lb_parQdrtIndc^2)));
      | lb_iQdrtCurrFWLim = sqrt(lb_parMaxPhsCurr^2 - lb_iQdrtCurrFWLim^2);
  lb_mfPermMagFlux : Inport
  lb_wActElctSpd : Inport  Port=2
  lb_vtEfcMaxVoltAmp : Inport  Port=3
  lb_iDmgzDirCurr : Inport  Port=4
  Add12 : Sum  OutDataTypeStr=Inherit: Same as first input
  Add13 : Sum  Inputs=+-  OutDataTypeStr=Inherit: Inherit via back propagation
  Add14 : Sum  Inputs=+-  OutDataTypeStr=Inherit: Same as first input
  Add8 : Sum  Inputs=+-  OutDataTypeStr=Inherit: Inherit via back propagation
  Add9 : Sum  Inputs=++-  OutDataTypeStr=Inherit: Inherit via back propagation
  Constant : Constant  Value=0  OutDataTypeStr=Inherit: Inherit via back propagation
  Constant1 : Constant  Value=lb_parMaxPhsCurr
  Constant11 : Constant  Value=lb_parQdrtIndc
  Constant12 : Constant  Value=lb_parDirIndc
  Constant13 : Constant  Value=lb_parDirIndc
  Constant14 : Constant  Value=lb_parQdrtIndc
  Constant15 : Constant  Value=lb_parMaxPhsCurr
  Constant20 : Constant  Value=lb_parMaxPhsCurr
  Data Type Duplicate : DataTypeDuplicate
  Data Type Duplicate1 : DataTypeDuplicate  NumInputPorts=3
  Data Type Duplicate2 : DataTypeDuplicate  NumInputPorts=3
  Data Type Conversion : DataTypeConversion  SaturateOnIntegerOverflow=off  RndMeth=Floor
  Divide3 : Product  Inputs=*/  OutDataTypeStr=Inherit: Inherit via back propagation
  Divide4 : Product  Inputs=*/  OutDataTypeStr=Inherit: Inherit via back propagation
  Divide5 : Product  Inputs=*/  OutDataTypeStr=Inherit: Inherit via back propagation
  Gain : Gain  Gain=-1  OutDataTypeStr=Inherit: Same as input
  Max : MinMax  Function=max  Inputs=2  OutDataTypeStr=Inherit: Inherit via back propagation
  Product2 : Product  OutDataTypeStr=Inherit: Inherit via back propagation
  Product3 : Product  OutDataTypeStr=Inherit: Inherit via back propagation
  Square{6..11,14..15} (8 alike) : Math  Operator=square  SignedPower=on  OutDataTypeStr=Inherit: Inherit via back propagation
  lib_Conversion_2 : lib_conversion/lib_Conversion_0  lb_parDataType=Inherit: Inherit via back propagation  lb_parOutpMaxVal=[]  lb_parOutpMinVal=[]  lb_parSatFlag=off
  lib_DynamicSaturator_1 : lib_dynamic_saturator/lib_DynamicSaturator_0
  lib_SquareRoot_1 : lib_square_root/lib_SquareRoot_0  lb_parLktSize=128  lb_parInpDataType=uint16  lb_parOutpDataType=Inherit: Inherit via back propagation
  lib_SquareRoot_2 : lib_square_root/lib_SquareRoot_0  lb_parLktSize=128  lb_parInpDataType=uint16  lb_parOutpDataType=Inherit: Inherit via back propagation
  lib_s16p27b0_1 : lib_conversion/lib_Conversion_0  lb_parDataType=fixdt(1,16,2^-27,0)  lb_parOutpMaxVal=[]  lb_parOutpMinVal=[]  lb_parSatFlag=off
  lib_s16p35b0_1 : lib_conversion/lib_Conversion_0  lb_parDataType=fixdt(1,16,2^-35,0)  lb_parOutpMaxVal=[]  lb_parOutpMinVal=[]  lb_parSatFlag=off
  lib_s16p5b0_1 : lib_conversion/lib_Conversion_0  lb_parDataType=fixdt(1,16,2^-5,0)  lb_parOutpMaxVal=[]  lb_parOutpMinVal=[]  lb_parSatFlag=off
  lib_s16p5b0_2 : lib_conversion/lib_Conversion_0  lb_parDataType=fixdt(1,16,2^-5,0)  lb_parOutpMaxVal=[]  lb_parOutpMinVal=[]  lb_parSatFlag=off
  lib_s32p13b0_1 : lib_conversion/lib_Conversion_0  lb_parDataType=fixdt(1,32,2^-13,0)  lb_parOutpMaxVal=[]  lb_parOutpMinVal=[]  lb_parSatFlag=off
  lib_u16p0b0_3 : lib_conversion/lib_Conversion_0  lb_parDataType=uint16  lb_parOutpMaxVal=[]  lb_parOutpMinVal=[]  lb_parSatFlag=off
  lib_u16p18b0_1 : lib_conversion/lib_Conversion_0  lb_parDataType=fixdt(0,16,2^-18,0)  lb_parOutpMaxVal=[]  lb_parOutpMinVal=[]  lb_parSatFlag=off
  lib_u16p18b0_2 : lib_conversion/lib_Conversion_0  lb_parDataType=fixdt(0,16,2^-18,0)  lb_parOutpMaxVal=[]  lb_parOutpMinVal=[]  lb_parSatFlag=off
  lib_u16p28b0_{1..4} (4 alike) : lib_conversion/lib_Conversion_0  lb_parDataType=fixdt(0,16,2^-28,0)  lb_parOutpMaxVal=[]  lb_parOutpMinVal=[]  lb_parSatFlag=off
  lib_u16p36b0_1 : lib_conversion/lib_Conversion_0  lb_parDataType=fixdt(0,16,2^-36,0)  lb_parOutpMaxVal=[]  lb_parOutpMinVal=[]  lb_parSatFlag=off
  lib_u16p36b0_2 : lib_conversion/lib_Conversion_0  lb_parDataType=fixdt(0,16,2^-36,0)  lb_parOutpMaxVal=[]  lb_parOutpMinVal=[]  lb_parSatFlag=off
  lib_u16p4b0_4 : lib_conversion/lib_Conversion_0  lb_parDataType=fixdt(0,16,2^-4,0)  lb_parOutpMaxVal=[]  lb_parOutpMinVal=[]  lb_parSatFlag=off
  lib_u32p14b0_2 : lib_conversion/lib_Conversion_0  lb_parDataType=fixdt(0,32,2^-14,0)  lb_parOutpMaxVal=[]  lb_parOutpMinVal=[]  lb_parSatFlag=off
  lb_iDirCurrFWLim : Outport
  lb_iQdrtCurrFWLim : Outport  Port=2
  wires:
  Constant14/1 -> Product3/1
  Product2/1 -> lib_u16p28b0_1/1
  Add8/1 -> lib_s16p35b0_1/1
  Divide3/1 -> Square8/1, lib_s16p5b0_1/1
  Constant15/1 -> Product3/2
  Add12/1 -> lib_SquareRoot_1/1
  Constant13/1 -> Product2/2
  [lb_vtEfcMaxVoltAmp] -> Divide4/1
  Constant11/1 -> Square6/1
  lib_s16p5b0_1/1 -> Add13/1
  [lb_iDirCurrFWLim] -> Square14/1
  Square8/1 -> lib_u32p14b0_2/1
  Add9/1 -> lib_s16p27b0_1/1
  Add14/1 -> lib_SquareRoot_2/1
  Square14/1 -> lib_u16p4b0_4/1
  Constant20/1 -> Square15/1
  Square15/1 -> lib_u16p0b0_3/1
  lib_SquareRoot_1/1 -> lib_s16p5b0_2/1
  lb_mfPermMagFlux/1 -> [lb_mfPermMagFlux]
  [lb_mfPermMagFlux] -> Product2/1
  [lb_mfPermMagFlux] -> Square9/1
  lb_wActElctSpd/1 -> [lb_wActElctSpd]
  [lb_wActElctSpd] -> Divide4/2
  [lb_iDirCurrFWLim] -> lb_iDirCurrFWLim/1
  lib_SquareRoot_2/1 -> [lb_iQdrtCurrFWLim]
  [lb_iQdrtCurrFWLim] -> lb_iQdrtCurrFWLim/1
  lib_u16p28b0_1/1 -> Divide3/1
  lib_u16p36b0_2/1 -> Add8/1
  lib_u16p36b0_1/1 -> Add8/2
  lib_s16p35b0_1/1 -> [lb_parSqrdIndcDiff], Divide3/2
  lib_u16p28b0_2/1 -> Add9/1
  Product3/1 -> lib_u16p18b0_1/1
  lib_u16p18b0_1/1 -> Square10/1
  Square10/1 -> lib_u16p28b0_3/1
  lib_u16p28b0_3/1 -> Add9/2
  Square9/1 -> lib_u16p28b0_2/1
  Divide4/1 -> lib_u16p18b0_2/1
  lib_u16p18b0_2/1 -> Square11/1
  Square11/1 -> lib_u16p28b0_4/1
  lib_u16p28b0_4/1 -> Add9/3
  lib_s16p27b0_1/1 -> Divide5/1
  [lb_parSqrdIndcDiff] -> Divide5/2
  lib_u32p14b0_2/1 -> Add12/1
  Divide5/1 -> lib_s32p13b0_1/1
  lib_s32p13b0_1/1 -> Add12/2
  lib_s16p5b0_2/1 -> Add13/2
  lib_u16p0b0_3/1 -> Add14/1
  lib_u16p4b0_4/1 -> Add14/2
  Square7/1 -> lib_u16p36b0_1/1
  Constant12/1 -> Square7/1
  Square6/1 -> lib_u16p36b0_2/1
  Add13/1 -> Data Type Duplicate1/3, lib_DynamicSaturator_1/2
  lib_DynamicSaturator_1/1 -> [lb_iDirCurrFWLim]
  lib_Conversion_2/1 -> Data Type Duplicate1/1, lib_DynamicSaturator_1/1
  Constant/1 -> lib_Conversion_2/1
  [lb_iDirCurrFWLim] -> Data Type Duplicate1/2
  lb_vtEfcMaxVoltAmp/1 -> [lb_vtEfcMaxVoltAmp]
  lb_iDmgzDirCurr/1 -> [lb_iDmgzDirCurr]
  Constant1/1 -> Data Type Conversion/1
  Gain/1 -> Max/2
  Data Type Conversion/1 -> Data Type Duplicate2/1, Gain/1
  [lb_iDirCurrFWLim] -> Data Type Duplicate2/3
  [lb_iDmgzDirCurr] -> Data Type Duplicate2/2
  [lb_iDmgzDirCurr] -> Max/1
  Max/1 -> [lb_iDirCurrFWLowLim]
  [lb_iDirCurrFWLowLim] -> Data Type Duplicate/1, lib_DynamicSaturator_1/3
  [lb_iDirCurrFWLim] -> Data Type Duplicate/2

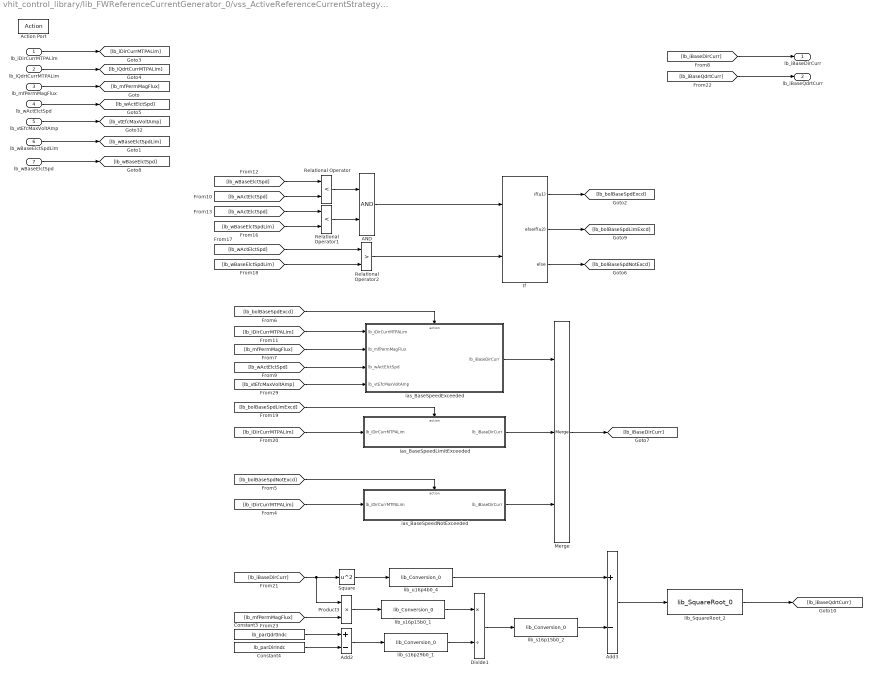
== system vhit_control_library/lib_FWReferenceCurrentGenerator_0/vss_ActiveReferenceCurrentStrategy/vss_FieldWeakeningStrategy/sss_BaseSpeedComputation/ias_CurrentMTPALimitAsymmetricMotorCondition ==
  lb_iDirCurrMTPALim : Inport
  lb_iQdrtCurrMTPALim : Inport  Port=2
  lb_mfPermMagFlux : Inport  Port=3
  lb_wActElctSpd : Inport  Port=4
  lb_vtEfcMaxVoltAmp : Inport  Port=5
  lb_wBaseElctSpdLim : Inport  Port=6
  lb_wBaseElctSpd : Inport  Port=7
  Action Port : ActionPort
  AND : Logic  AllPortsSameDT=off  OutDataTypeStr=boolean
  Add2 : Sum  Inputs=+-  OutDataTypeStr=Inherit: Inherit via back propagation
  Add3 : Sum  Inputs=+-  OutDataTypeStr=Inherit: Same as first input
  Constant3 : Constant  Value=lb_parQdrtIndc
  Constant4 : Constant  Value=lb_parDirIndc
  Divide1 : Product  Inputs=*/  OutDataTypeStr=Inherit: Inherit via back propagation
  If : If  NumInputs=2  IfExpression=u1  ElseIfExpressions=u2
  Merge : Merge  Inputs=3
  Product3 : Product  OutDataTypeStr=Inherit: Inherit via back propagation
  Relational Operator : RelationalOperator  Operator=<  OutDataTypeStr=boolean  RndMeth=Simplest  InputSameDT=off
  Relational Operator1 : RelationalOperator  Operator=<  OutDataTypeStr=boolean  RndMeth=Simplest  InputSameDT=off
  Relational Operator2 : RelationalOperator  Operator=>  OutDataTypeStr=boolean  RndMeth=Simplest  InputSameDT=off
  Square : Math  Operator=square  SignedPower=on  OutDataTypeStr=Inherit: Inherit via back propagation
  ias_BaseSpeedExceeded : Subsystem  TreatAsAtomicUnit=on
  ias_BaseSpeedLimitExceeded : Subsystem  TreatAsAtomicUnit=on
  ias_BaseSpeedNotExceeded : Subsystem  TreatAsAtomicUnit=on
  lib_SquareRoot_2 : lib_square_root/lib_SquareRoot_0  lb_parLktSize=128  lb_parInpDataType=uint16  lb_parOutpDataType=Inherit: Inherit via back propagation
  lib_s16p15b0_1 : lib_conversion/lib_Conversion_0  lb_parDataType=fixdt(1,16,2^-15,0)  lb_parOutpMaxVal=[]  lb_parOutpMinVal=[]  lb_parSatFlag=off
  lib_s16p15b0_2 : lib_conversion/lib_Conversion_0  lb_parDataType=fixdt(1,16,2^-3,0)  lb_parOutpMaxVal=[]  lb_parOutpMinVal=[]  lb_parSatFlag=off
  lib_s16p29b0_1 : lib_conversion/lib_Conversion_0  lb_parDataType=fixdt(1,16,2^-29,0)  lb_parOutpMaxVal=[]  lb_parOutpMinVal=[]  lb_parSatFlag=off
  lib_u16p4b0_4 : lib_conversion/lib_Conversion_0  lb_parDataType=fixdt(0,16,2^-4,0)  lb_parOutpMaxVal=[]  lb_parOutpMinVal=[]  lb_parSatFlag=off
  lb_iBaseDirCurr : Outport
  lb_iBaseQdrtCurr : Outport  Port=2
  wires:
  lb_wBaseElctSpd/1 -> [lb_wBaseElctSpd]
  lb_wBaseElctSpdLim/1 -> [lb_wBaseElctSpdLim]
  [lb_iBaseDirCurr] -> lb_iBaseDirCurr/1
  [lb_iBaseQdrtCurr] -> lb_iBaseQdrtCurr/1
  lb_vtEfcMaxVoltAmp/1 -> [lb_vtEfcMaxVoltAmp]
  lb_mfPermMagFlux/1 -> [lb_mfPermMagFlux]
  lb_wActElctSpd/1 -> [lb_wActElctSpd]
  lb_iDirCurrMTPALim/1 -> [lb_iDirCurrMTPALim]
  lb_iQdrtCurrMTPALim/1 -> [lb_iQdrtCurrMTPALim]
  [lb_wBaseElctSpd] -> Relational Operator/1
  [lb_iDirCurrMTPALim] -> ias_BaseSpeedExceeded/1(lb_iDirCurrMTPALim)
  Add3/1 -> lib_SquareRoot_2/1
  lib_SquareRoot_2/1 -> [lb_iBaseQdrtCurr]
  [lb_wActElctSpd] -> Relational Operator2/1
  [lb_mfPermMagFlux] -> ias_BaseSpeedExceeded/2(lb_mfPermMagFlux)
  [lb_wActElctSpd] -> Relational Operator/2
  Product3/1 -> lib_s16p15b0_1/1
  [lb_vtEfcMaxVoltAmp] -> ias_BaseSpeedExceeded/4(lb_vtEfcMaxVoltAmp)
  Constant4/1 -> Add2/2
  Constant3/1 -> Add2/1
  If/3 -> [lb_bolBaseSpdNotExcd]
  [lb_iDirCurrMTPALim] -> ias_BaseSpeedLimitExceeded/1(lb_iDirCurrMTPALim)
  ias_BaseSpeedNotExceeded/1(lb_iBaseDirCurr) -> Merge/3
  AND/1 -> If/1
  [lb_iBaseDirCurr] -> Product3/1, Square/1
  [lb_wBaseElctSpdLim] -> Relational Operator1/2
  Relational Operator2/1 -> If/2
  Square/1 -> lib_u16p4b0_4/1
  lib_s16p15b0_1/1 -> Divide1/1
  Relational Operator/1 -> AND/1
  [lb_wActElctSpd] -> Relational Operator1/1
  lib_s16p15b0_2/1 -> Add3/2
  Divide1/1 -> lib_s16p15b0_2/1
  lib_s16p29b0_1/1 -> Divide1/2
  [lb_mfPermMagFlux] -> Product3/2
  lib_u16p4b0_4/1 -> Add3/1
  Add2/1 -> lib_s16p29b0_1/1
  [lb_wBaseElctSpdLim] -> Relational Operator2/2
  ias_BaseSpeedLimitExceeded/1(lb_iBaseDirCurr) -> Merge/2
  [lb_bolBaseSpdLimExcd] -> ias_BaseSpeedLimitExceeded/Action
  [lb_bolBaseSpdNotExcd] -> ias_BaseSpeedNotExceeded/Action
  [lb_iDirCurrMTPALim] -> ias_BaseSpeedNotExceeded/1(lb_iDirCurrMTPALim)
  Merge/1 -> [lb_iBaseDirCurr]
  [lb_bolBaseSpdExcd] -> ias_BaseSpeedExceeded/Action
  ias_BaseSpeedExceeded/1(lb_iBaseDirCurr) -> Merge/1
  If/1 -> [lb_bolBaseSpdExcd]
  [lb_wActElctSpd] -> ias_BaseSpeedExceeded/3(lb_wActElctSpd)
  If/2 -> [lb_bolBaseSpdLimExcd]
  Relational Operator1/1 -> AND/2

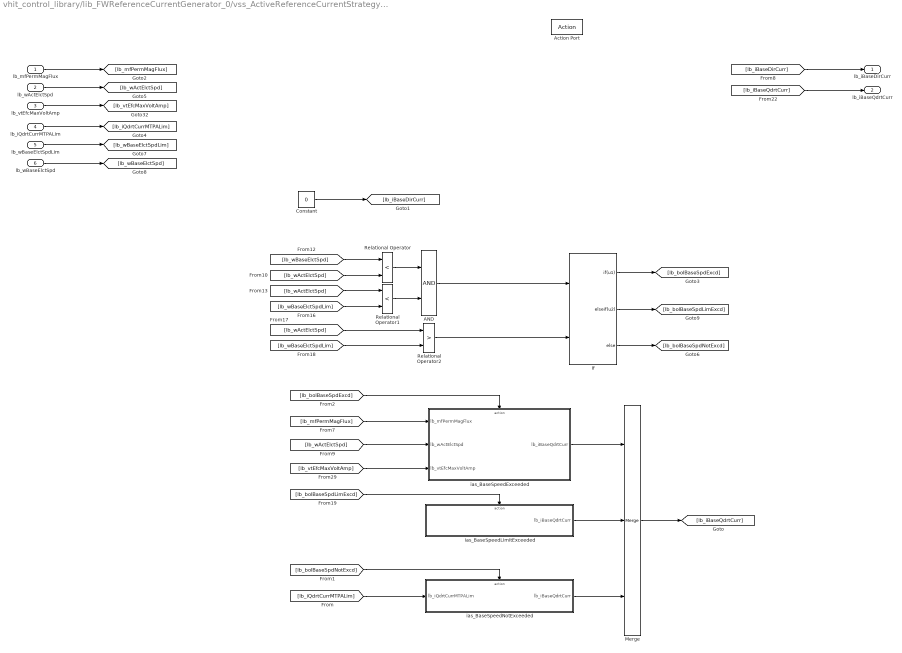
== system vhit_control_library/lib_FWReferenceCurrentGenerator_0/vss_ActiveReferenceCurrentStrategy/vss_FieldWeakeningStrategy/sss_BaseSpeedComputation/ias_CurrentMTPALimitSymmetricMotorCondition ==
  lb_mfPermMagFlux : Inport
  lb_wActElctSpd : Inport  Port=2
  lb_vtEfcMaxVoltAmp : Inport  Port=3
  lb_iQdrtCurrMTPALim : Inport  Port=4
  lb_wBaseElctSpdLim : Inport  Port=5
  lb_wBaseElctSpd : Inport  Port=6
  Action Port : ActionPort
  AND : Logic  AllPortsSameDT=off  OutDataTypeStr=boolean
  Constant : Constant  Value=0  OutDataTypeStr=Inherit: Inherit via back propagation
  If : If  NumInputs=2  IfExpression=u1  ElseIfExpressions=u2
  Merge : Merge  Inputs=3
  Relational Operator : RelationalOperator  Operator=<  OutDataTypeStr=boolean  RndMeth=Simplest  InputSameDT=off
  Relational Operator1 : RelationalOperator  Operator=<  OutDataTypeStr=boolean  RndMeth=Simplest  InputSameDT=off
  Relational Operator2 : RelationalOperator  Operator=>  OutDataTypeStr=boolean  RndMeth=Simplest  InputSameDT=off
  ias_BaseSpeedExceeded : Subsystem  TreatAsAtomicUnit=on
  ias_BaseSpeedLimitExceeded : Subsystem  TreatAsAtomicUnit=on
  ias_BaseSpeedNotExceeded : Subsystem  TreatAsAtomicUnit=on
  lb_iBaseDirCurr : Outport
  lb_iBaseQdrtCurr : Outport  Port=2
  wires:
  lb_wBaseElctSpd/1 -> [lb_wBaseElctSpd]
  lb_wBaseElctSpdLim/1 -> [lb_wBaseElctSpdLim]
  [lb_iQdrtCurrMTPALim] -> ias_BaseSpeedNotExceeded/1(lb_iQdrtCurrMTPALim)
  lb_iQdrtCurrMTPALim/1 -> [lb_iQdrtCurrMTPALim]
  Constant/1 -> [lb_iBaseDirCurr]
  [lb_wBaseElctSpdLim] -> Relational Operator1/2
  If/3 -> [lb_bolBaseSpdNotExcd]
  [lb_wActElctSpd] -> Relational Operator1/1
  [lb_wActElctSpd] -> ias_BaseSpeedExceeded/2(lb_wActElctSpd)
  ias_BaseSpeedExceeded/1(lb_iBaseQdrtCurr) -> Merge/1
  Relational Operator2/1 -> If/2
  Relational Operator/1 -> AND/1
  [lb_mfPermMagFlux] -> ias_BaseSpeedExceeded/1(lb_mfPermMagFlux)
  ias_BaseSpeedNotExceeded/1(lb_iBaseQdrtCurr) -> Merge/3
  AND/1 -> If/1
  [lb_wActElctSpd] -> Relational Operator2/1
  ias_BaseSpeedLimitExceeded/1(lb_iBaseQdrtCurr) -> Merge/2
  [lb_wBaseElctSpd] -> Relational Operator/1
  [lb_vtEfcMaxVoltAmp] -> ias_BaseSpeedExceeded/3(lb_vtEfcMaxVoltAmp)
  [lb_wActElctSpd] -> Relational Operator/2
  [lb_wBaseElctSpdLim] -> Relational Operator2/2
  [lb_bolBaseSpdExcd] -> ias_BaseSpeedExceeded/Action
  Merge/1 -> [lb_iBaseQdrtCurr]
  [lb_bolBaseSpdNotExcd] -> ias_BaseSpeedNotExceeded/Action
  [lb_bolBaseSpdLimExcd] -> ias_BaseSpeedLimitExceeded/Action
  If/1 -> [lb_bolBaseSpdExcd]
  Relational Operator1/1 -> AND/2
  If/2 -> [lb_bolBaseSpdLimExcd]
  lb_vtEfcMaxVoltAmp/1 -> [lb_vtEfcMaxVoltAmp]
  lb_wActElctSpd/1 -> [lb_wActElctSpd]
  lb_mfPermMagFlux/1 -> [lb_mfPermMagFlux]
  [lb_iBaseQdrtCurr] -> lb_iBaseQdrtCurr/1
  [lb_iBaseDirCurr] -> lb_iBaseDirCurr/1
